simulink model "modello_motore_PID_desaturatore"  (R2014b)
settings: Solver=ode45  StartTime=0.0  StopTime=10.0  RelTol=1e-3
values from neighbouring files (symbols this model uses):
  d = 0    [controllo_motore_stato.m]    (also in controllo_motore_stato_integrale.m = -0.2; modello_motore.m = 0.5)
  K_a = 1 / (3 * t_s_max * K_i)    [modello_motore.m]
  K_d = K_p^2 / (b * K_i)    [modello_motore.m]
  K_g2v = 0.0284    [modello_motore.m]
  K_i = ((a * w_a_min) / 2) * (sqrt((sin(theta))^2 +      (4/b)*(cos(theta))^2) - sin(theta))    [modello_motore.m]
  K_p = a * cos(theta)    [modello_motore.m]
  K_r2v = 1.63    [modello_motore.m]
  r = 50    [controllo_motore_stato.m]    (also in controllo_motore_stato_integrale.m = 120; modello_motore.m = 10)
  tau_L = alpha / w_a_min    (= 0.007)    [modello_motore.m]
undefined symbols (not defined in the file or in its folder): denP, numP
settings Model: Creator=Nicola  LastModifiedBy=Nicola
settings SolverCC: AutoInsertRateTranBlk=on
settings DataIOCC: SaveOutput=off  SaveTime=off
settings OptimizationCC: InlineParams=on  InlineInvariantSignals=on  StateBitsets=on  DataBitsets=on  UseTempVars=on  ZeroExternalMemoryAtStartup=off  ZeroInternalMemoryAtStartup=off  NoFixptDivByZeroProtection=on  OptimizeModelRefInitCode=on  LifeSpan=1
settings DebuggingCC: UnderspecifiedInitializationDetection=Classic  MergeDetectMultiDrivingBlocksExec=none  StateNameClashWarn=warning
settings HardwareCC: ProdIntDivRoundTo=Floor  ProdEndianess=LittleEndian  ProdHWDeviceType=Generic->Custom
settings RTWCC: SystemTargetFile=ert.tlc  TLCOptions=-p0  GenCodeOnly=on  TemplateMakefile=ert_default_tmf  Description=Embedded Coder  GenerateReport=on  RTWVerbose=off  ProcessScript=ert_make_rtw_hook  IncludeHyperlinkInReport=on  LaunchReport=on
settings CodeAppCC: ForceParamTrailComments=on  IgnoreCustomStorageClasses=off  SimulinkDataObjDesc=on  CustomSymbolStrGlobalVar=rt$N$M  CustomSymbolStrType=$N$M  CustomSymbolStrFcn=$N$M$F  CustomSymbolStrMacro=$N$M  InsertBlockDesc=on
settings ERTTargetCC: TargetLangStandard=C99 (ISO)  GenerateSampleERTMain=on  IncludeMdlTerminateFcn=off  SuppressErrorStatus=on  SupportAbsoluteTime=off  SupportNonFinite=off  SupportComplex=off  PurelyIntegerCode=on  InlinedParameterPlacement=NonHierarchical  RootIOFormat=Structure reference  ERTCustomFileTemplate=example_file_process.tlc

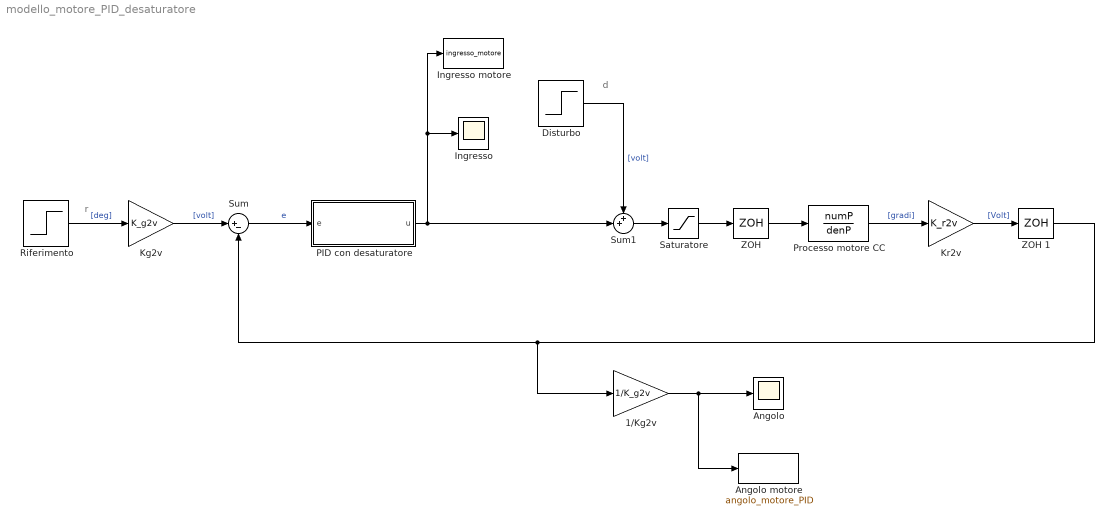
== system modello_motore_PID_desaturatore ==
  note: d
  note: r
  "1/Kg2v " : Gain  Gain=1/K_g2v
  Angolo : Scope
  Angolo motore : ToWorkspace  VariableName=angolo_motore_PID  SampleTime=-1
  Disturbo : Step  After=d  SampleTime=0
  Ingresso : Scope
  Ingresso motore : ToWorkspace  VariableName=ingresso_motore  SampleTime=-1
  Kg2v : Gain  Gain=K_g2v
  Kr2v : Gain  Gain=K_r2v
  PID con desaturatore : Subsystem
  Processo motore CC : TransferFcn  Numerator=numP  Denominator=denP
  Riferimento : Step  After=r  SampleTime=0
  "Saturatore " : Saturate  UpperLimit=5  LowerLimit=-5
  Sum : Sum  Inputs=|+-
  Sum1 : Sum  Inputs=++|
  ZOH : ZeroOrderHold  SampleTime=0.001
  "ZOH 1 " : ZeroOrderHold  SampleTime=0.001
  wires:
  Riferimento/1 -> Kg2v/1  "[deg]"
  Kg2v/1 -> Sum/1  "[volt]"
  "Saturatore "/1 -> ZOH/1
  ZOH/1 -> Processo motore CC/1
  Processo motore CC/1 -> Kr2v/1  "[gradi]"
  Kr2v/1 -> "ZOH 1 "/1  "[Volt]"
  "ZOH 1 "/1 -> "1/Kg2v "/1, Sum/2
  "1/Kg2v "/1 -> Angolo motore/1, Angolo/1
  Sum/1 -> PID con desaturatore/1(e)  "e"
  PID con desaturatore/1(u) -> Sum1/2, Ingresso/1, Ingresso motore/1
  Sum1/1 -> "Saturatore "/1
  Disturbo/1 -> Sum1/1  "[volt]"

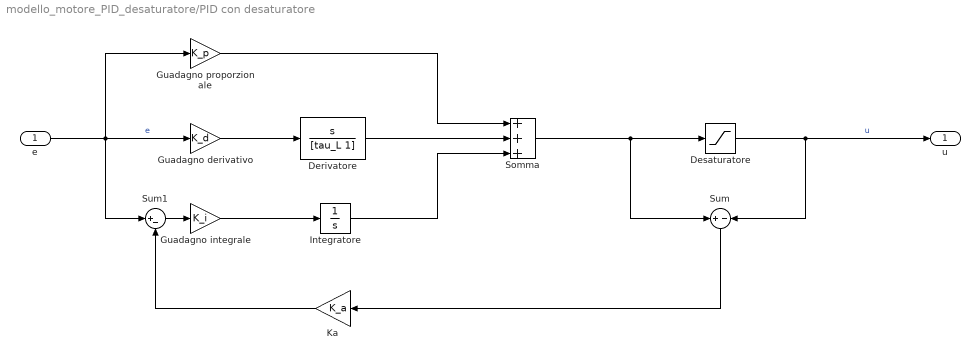
== system modello_motore_PID_desaturatore/PID con desaturatore ==
  e : Inport
  Derivatore : TransferFcn  Numerator=[1 0]  Denominator=[tau_L 1]
  "Desaturatore " : Saturate  UpperLimit=5  LowerLimit=-5
  Guadagno derivativo : Gain  Gain=K_d
  Guadagno integrale : Gain  Gain=K_i
  Guadagno proporzionale : Gain  Gain=K_p
  Integratore : Integrator
  Ka : Gain  Gain=K_a
  Somma : Sum  Inputs=3  SaturateOnIntegerOverflow=on  InputSameDT=on  OutDataTypeStr=Inherit: Same as first input
  Sum : Sum  Inputs=+-
  Sum1 : Sum  Inputs=|+-
  u : Outport
  wires:
  e/1 -> Guadagno proporzionale/1, Sum1/1, Guadagno derivativo/1  "e"
  Guadagno derivativo/1 -> Derivatore/1
  Derivatore/1 -> Somma/2
  Integratore/1 -> Somma/3
  Guadagno proporzionale/1 -> Somma/1
  "Desaturatore "/1 -> Sum/2, u/1  "u"
  Somma/1 -> "Desaturatore "/1, Sum/1
  Ka/1 -> Sum1/2
  Guadagno integrale/1 -> Integratore/1
  Sum1/1 -> Guadagno integrale/1
  Sum/1 -> Ka/1
